simulink library "socmemlib"  (R2021a)
settings: Solver=VariableStepAuto  StartTime=0.0  StopTime=10.0  RelTol=1e-3
PreLoadFcn:
  | soc.internal.HWSWMessageTypeDef();
  | hsb.blkcb2.defineTypes;
undefined symbols (not defined in the file or in its folder): BurstRequest2BusObj, gcbh, hsb, m, ReadAccessBusObj, rearb, RegA, sendFifoFreeMsg, soc, WriteAccessBusObj
libraries: socmemlib_internal x59, priv_hsblib_beta2 x34, socsharedlib_internal x2, socqueuelib_internal x1, simulink x1
(part 4 of 5)

== stateflow chart socmemlib/Memory Channel/Writer 1/To Memory Channel/Addressable To Memory Channel/Addressable Channel Write Slave Interface/A4M Wr Slave BFM ==
  settings: updateMethod=DISCRETE  sampleTime=ChFrameSampleTime  enableNonTerminalStates=1
  state fullchart
    state requestPipeline [parallel]
      settings: executionOrder=2
      state waitForTransaction
        entry:
        wrCtrlS2M.wr_ready = true;
      state queueTransaction
        entry:
        checkAddressRange(double(wrCtrlM2S.wr_addr),double(wrCtrlM2S.wr_len), ...
        MRRegionSize,'Writer',ChTDATAWidth);
        FIFOChGatherCount = wrCtrlM2S.wr_len/ChLength;
        ReqFIFO.data = wrCtrlM2S;
        send(ReqFIFO);
        transInFlight = transInFlight +1;
      state waitForValid
      state readyTrue
        entry:
        wrCtrlS2M.wr_ready = true;
      state queueData
        entry:
        DataFIFO.data = packDataIn;
        send(DataFIFO);
        dataInFlight = dataInFlight +1;
        FIFOGatheredCount = FIFOGatheredCount+1;
      state waitForDataFIFO
      state waitFor1cycle
      state readyFalse1
        entry:
        wrCtrlS2M.wr_ready = false;
      state readyFalse
        entry:
        wrCtrlS2M.wr_ready = false;
      state queueLastData
        entry:
        if (wrCtrlM2S.wr_valid == true) && ...
        (dataInFlight<PipelineDepth+1)
        DataFIFO.data = packDataIn;
        send(DataFIFO);
        dataInFlight = dataInFlight +1;
        FIFOGatheredCount = FIFOGatheredCount+1;
        end
      state waitForFIFOs
      (default) -> waitForTransaction
      waitForFIFOs -> waitForTransaction : [(transInFlight<PipelineDepth) && ...
          |  (dataInFlight<PipelineDepth)]
      waitFor1cycle -> waitForTransaction [order 2] : after(ChFrameSampleTime, sec)
      waitForTransaction -> queueTransaction : [wrCtrlM2S.wr_valid == true]
      waitForValid -> queueData : [wrCtrlM2S.wr_valid == true]
      readyTrue -> waitForValid : after(ChFrameSampleTime, sec)
      queueTransaction -> queueData : {FIFOGatheredCount = 0;}
      queueData -> readyTrue [order 3]
      waitForDataFIFO -> readyTrue : [dataInFlight<PipelineDepth]
      queueData -> waitFor1cycle [order 1] : [(FIFOGatheredCount == FIFOChGatherCount)]
      queueData -> readyFalse1 [order 2] : [~(dataInFlight<PipelineDepth)]
      queueLastData -> waitFor1cycle [order 1] : [(FIFOGatheredCount == FIFOChGatherCount)]
      queueLastData -> waitForDataFIFO [order 2]
      waitFor1cycle -> readyFalse [order 1] : [~((transInFlight<PipelineDepth) && ...
          |  (dataInFlight<PipelineDepth))]
      readyFalse1 -> queueLastData : after(ChFrameSampleTime, sec)
      readyFalse -> waitForFIFOs : after(ChFrameSampleTime, sec)
    state initVars [parallel]
      settings: executionOrder=1
      state init
        entry:
        wrCtrlS2M = struct('wr_ready', true, 'wr_bvalid', false, 'wr_complete', false);
        locBData = zeros(4096,1,'uint8'); % FIXME: 4096 is absolute max size; MaximumBurstSize reflects tdata/len
        gatherBuffer = zeros(ChGatherBufferSize, 1, 'uint8');
        gatherBufferIndex = 1;
        burstsInFlight = 0;
        transInFlight = 0;
        dataInFlight = 0;
        frameDone = false;
      (default) -> fullchart.initVars.init
    state sendRequests [parallel]
      settings: executionOrder=3
      state waitForReq
        entry:
      state addrAndFirstData
        entry:
        CurrReq = ReqFIFO.data;
        locBAddr = double(CurrReq.wr_addr);
        [locChGatherCount, nthBSize, locChGatherBufferBurstCount] = ...
        calcDerivedInfo(double(CurrReq.wr_len), ChLength, ChTDATAWidth, ...
        ChFrameGatherBufferSize,  ChGatherBufferSize);
      state gather
        entry:
        CurrData = DataFIFO.data;
        gatheredCount = gatheredCount+1;
        gatherBuffer(gatherBufferIndex:gatherBufferIndex+ChFrameGatherBufferSize-1) = CurrData;
        gatherBufferIndex = gatherBufferIndex + ChFrameGatherBufferSize;
        dataInFlight = dataInFlight - 1;
      state waitForData
      state waitForAllBurstsToComplete
      note: If we are at the last burst OR we have enough data for one or more max-sized bursts
      state createBurst
        entry:
        if sentBurstCount == (locChGatherBufferBurstCount-1)
        currBSize = nthBSize;
        else
        currBSize = MaximumBurstSize;
        end
        burstNum = burstNum+1;
        locBData(1:currBSize) = gatherBuffer(sentBufferIndex:sentBufferIndex+currBSize-1);
      state sendBurst
        entry:
        writeToMem.data = struct('accessID', burstNum, ...
        'addr', locBAddr, 'size', currBSize,  ...
        'wdata', locBData, 'bufferAction', BufferAction.none);
        send(writeToMem);
        sentBufferIndex = sentBufferIndex + currBSize;
        locBAddr = locBAddr + currBSize;
        sentBurstCount = sentBurstCount+1;
        burstsInFlight = burstsInFlight + 1;
        if sentBurstCount == locChGatherBufferBurstCount
        frameDone=true;
        end
      (default) -> waitForReq
      waitForAllBurstsToComplete -> waitForReq : [burstsInFlight==0]
          | {transInFlight = transInFlight -1;}
      waitForReq -> addrAndFirstData : ReqFIFO
      addrAndFirstData -> gather : DataFIFO
          | { gatherBufferIndex = 1;sentBurstCount = 0; gatheredCount = 0; }
      waitForData -> gather : DataFIFO
      (junction 348) -> waitForAllBurstsToComplete [order 2] : [sentBurstCount == locChGatherBufferBurstCount]
      gather -> waitForData [order 2]
      (junction 348) -> waitForData [order 3] : [gatheredCount < locChGatherCount]
          | { gatherBufferIndex = 1;}
      gather -> createBurst [order 1] : [(gatheredCount == locChGatherCount) || (rem(gatherBufferIndex-1,MaximumBurstSize)==0)]
          | { sentBufferIndex = 1;}
      (junction 348) -> createBurst [order 1] : [sentBufferIndex < gatherBufferIndex]
      sendBurst -> (junction 348) : [burstsInFlight < InterconnectDepth]
      createBurst -> sendBurst : [memReady]
    state BurstsHandler [parallel]
      settings: executionOrder=4
      state init
        entry:
        wrCtrlS2M.wr_bvalid = false;
        wrCtrlS2M.wr_complete = false;
      state sendFrame
      state sendBursts
      state waitforFrameComplete
      state waitforBurstDone
        entry:
        wrCtrlS2M.wr_bvalid = false;
        wrCtrlS2M.wr_complete = true;
      state waitfor1Clock
      state writeIsDone
        entry:
        burstsInFlight=0;
        frameDone=false;
        wrCtrlS2M.wr_bvalid = true;
        wrCtrlS2M.wr_complete = true;
      state burstIsDone
        entry:
        if burstsInFlight >0
        wrCtrlS2M.wr_bvalid = true;
        burstsInFlight = burstsInFlight - 1;
        end
      state frameIsDone
        entry:
        if frameDone
        wrCtrlS2M.wr_complete = true;
        frameDone = false;
        end
      (default) -> fullchart.BurstsHandler.init
      (junction 413) -> fullchart.BurstsHandler.init [order 2]
      (junction 424) -> fullchart.BurstsHandler.init [order 2]
      fullchart.BurstsHandler.init -> sendFrame [order 1] : [frameDone && (ChLength>1)]
      fullchart.BurstsHandler.init -> sendBursts [order 2] : [burstsInFlight>0 || frameDone]
      (junction 424) -> waitforBurstDone [order 1] : [burstsInFlight>0]
      sendFrame -> waitforFrameComplete : after(ChFrameSampleTime,sec)
      sendBursts -> waitforBurstDone : after(ChFrameSampleTime,sec)
      waitfor1Clock -> waitforBurstDone : after(ChFrameSampleTime,sec)
      waitforFrameComplete -> writeIsDone : [memReady]
      waitforBurstDone -> burstIsDone : [memReady]
      frameIsDone -> (junction 424) : after(ChFrameSampleTime,sec)
      (junction 413) -> writeIsDone [order 1] : [frameDone && memReady]
      burstIsDone -> waitfor1Clock [order 1] : [burstsInFlight>0]
      writeIsDone -> (junction 413) : after(ChFrameSampleTime,sec)
      burstIsDone -> frameIsDone [order 2]
  (default) -> fullchart
  data: varargin function_input; varargout function_output; varargin function_input; packDataIn input; writeToMem output Bus: WriteAccessBusObj; wrCtrlS2M output Bus: WriteControlS2MBusObj; gatherBufferIndex local =1; burstNum local =0; gatherBuffer local; sentBurstCount local =0; gatheredCount local =0; locBData local uint8; ChFrameSampleTime parameter; locChGatherBufferBurstCount local; locChGatherCount local; ChFrameGatherBufferSize parameter; MaximumBurstSize parameter; ChLength parameter; ChTDATAWidth parameter; nthBSize local; locBAddr local; wrCtrlM2S input Bus: WriteControlM2SBusObj; ChGatherBufferSize parameter; memReady input; currBSize local; sentBufferIndex local; MRRegionSize parameter; PipelineDepth parameter; InterconnectDepth parameter; burstsInFlight local =0; ReqFIFO local Bus: WriteControlM2SBusObj; CurrReq local Bus: WriteControlM2SBusObj; DataFIFO local; CurrData local; FIFOChGatherCount local; FIFOGatheredCount local =0; transInFlight local =0; dataInFlight local =0; frameDone local =false
  function varargout = calcDerivedInfo(varargin):
    | function varargout = calcDerivedInfo(varargin)
    |     [varargout{1:nargout}] = hsb.blkcb2.PUPCodegenCb('calcDerivedInfo',varargin{:});
    | end
  function checkAddressRange(varargin):
    | function checkAddressRange(varargin)
    | 
    |     hsb.blkcb2.PUPCodegenCb('checkAddressRange',varargin{:});
    |     
    | end

== stateflow chart socmemlib/Memory Channel/Writer 1/To Memory Channel/Addressable To Memory Channel/Addressable Channel Write Slave Interface/Chart ==
  settings: updateMethod=DISCRETE  sampleTime=ChFrameSampleTime
  state init
    entry:
    readyDiscrete = true;
  state notvalid
    entry:
    readyDiscrete = false;
  (default) -> init
  notvalid -> init [order 1] : [readyFiM==true]
  init -> notvalid : [readyFiM==false]
  notvalid -> notvalid [order 2] : [readyFiM==false]
  data: readyFiM input; readyDiscrete output

== stateflow chart socmemlib/Memory Channel/Writer 1/To Memory Channel/Software Streaming To Memory Channel/Channel Streaming Slave Interface/A4S BFM ==
  settings: enableNonTerminalStates=1
  state fullchart
    state workChart [parallel]
      settings: executionOrder=1
      state init
        entry:
        gatherBuffer = zeros(ChGatherBufferSize, 1, 'uint8');
        bdata = zeros(MaximumBurstSize,1,'uint8');
      state requestBuffer
        entry:
        bdata = zeros(MaximumBurstSize,1,'uint8');
        MsgReqCtrl(); % Request a buffer
        writeToMem.data = struct('accessID', 0, 'addr', NO_INFLOW_DELAY, 'size', 0,  ...
        'wdata', bdata, 'bufferAction', BufferAction.request , ...
        'timingMode', TimingMode.untimed);
        send(writeToMem);
      state waitForEvent
      state gather
        entry:
        [packDataIn,valid] = MsgRecvCtrl();
        if valid
        gatheredCount = gatheredCount+1;
        gatherBuffer(gatherBufferIndex:gatherBufferIndex+ChFrameGatherBufferSize-1) = packDataIn;
        gatherBufferIndex = gatherBufferIndex + ChFrameGatherBufferSize;
        end
      state nextGather
      state sendBursts
        entry:
        reqAddr = NO_INFLOW_DELAY;
        burstNum = burstNum+1;
        bdata(1:BurstSize) = gatherBuffer(gatherBufferIndex:gatherBufferIndex+BurstSize-1);
        if sentBurstCount == ChGatherBufferBurstCount - 1;
        bufferAction = BufferAction.release;
        else
        bufferAction = BufferAction.none;
        end
        writeToMem.data = struct('accessID', burstNum, 'addr', reqAddr, 'size', BurstSize,  ...
        'wdata', bdata, 'bufferAction', bufferAction, 'timingMode', TimingMode.untimed);
        send(writeToMem);
        gatherBufferIndex = gatherBufferIndex + BurstSize;
        sentBurstCount = sentBurstCount+1;
      (default) -> init
      init -> requestBuffer
      nextGather -> requestBuffer [order 2]
      requestBuffer -> waitForEvent
      (junction 40) -> waitForEvent [order 2]
      waitForEvent -> gather : event
      nextGather -> gather [order 1] : event
      (junction 43) -> nextGather [order 1] : [sentBurstCount == ChGatherBufferBurstCount] { gatherBufferIndex = 1; sentBurstCount = 0; }
      gather -> (junction 40) : after(0,sec)
      (junction 40) -> sendBursts [order 1] : [gatheredCount == ChGatherCount] { gatherBufferIndex = 1; gatheredCount = 0; }
      (junction 43) -> sendBursts [order 2]
      sendBursts -> (junction 43) : after(0,sec)
  note: NOTE: Trying to use junctions instead
      | of state for 'nextGather' resulted in some
      | funky back-tracing where both transitions of
      | junction outputs were executed.
  (default) -> fullchart
  data: writeToMem output Bus: WriteAccessBusObj; packDataIn local; valid local boolean =false; bdata local uint8; burstNum local =0; BurstSize parameter; ChFrameGatherBufferSize parameter; ChGatherBufferBurstCount parameter; ChGatherBufferSize parameter; ChGatherCount parameter; gatherBuffer local; gatherBufferIndex local =1; gatheredCount local =0; MaximumBurstSize parameter; NO_INFLOW_DELAY constant double =-2; bufferAction local Enum: BufferAction; reqAddr local; sentBurstCount local =0; event input Bus: rteEvent

== stateflow chart socmemlib/Memory Channel/Writer 1/To Memory Channel/Streaming To Memory Channel/Channel Streaming Slave Interface/A4S BFM ==
  settings: updateMethod=DISCRETE  sampleTime=ChFrameSampleTime  enableNonTerminalStates=1
  state init
    entry:
    gatherBuffer = zeros(ChGatherBufferSize, 1, 'uint8');
    bdata = zeros(MaximumBurstSize,1,'uint8');
  state waitForValid
  state gather
    entry:
    gatheredCount = gatheredCount+1;
    gatherBuffer(gatherBufferIndex:gatherBufferIndex+ChFrameGatherBufferSize-1) = packDataIn;
    gatherBufferIndex = gatherBufferIndex + ChFrameGatherBufferSize;
  state nextGather
  state sendBursts
    entry:
    burstNum = burstNum+1;
    bdata(1:BurstSize) = gatherBuffer(gatherBufferIndex:gatherBufferIndex+BurstSize-1);
    if tlast
    bufferAction = BufferAction.release;
    else
    bufferAction = BufferAction.none;
    end
    writeToMem.data = struct('accessID', burstNum, 'addr', -1, 'size', BurstSize,  ...
    'wdata', bdata, 'bufferAction', bufferAction);
    send(writeToMem);
    gatherBufferIndex = gatherBufferIndex + BurstSize;
    sentBurstCount = sentBurstCount+1;
  (default) -> init
  init -> waitForValid
  nextGather -> waitForValid : after(ChFrameSampleTime, sec)
  waitForValid -> gather : [valid == true]
  gather -> nextGather [order 2]
  gather -> sendBursts [order 1] : [gatheredCount == ChGatherCount] { gatherBufferIndex = 1; gatheredCount = 0; }
  sendBursts -> nextGather [order 1] : [sentBurstCount == ChGatherBufferBurstCount] { gatherBufferIndex = 1; sentBurstCount = 0; }
  sendBursts -> sendBursts [order 2]
  data: packDataIn input; writeToMem output Bus: WriteAccessBusObj; valid input boolean; tlast input boolean; gatherBufferIndex local =1; burstNum local =0; gatherBuffer local; sentBurstCount local =0; gatheredCount local =0; bdata local uint8; BurstSize parameter; ChFrameSampleTime parameter; ChGatherBufferBurstCount parameter; ChGatherBufferSize parameter; ChGatherCount parameter; ChFrameGatherBufferSize parameter; MaximumBurstSize parameter; bufferAction local Enum: BufferAction

== stateflow chart socmemlib/Memory Channel/Writer 1/To Memory Channel/Streaming To Memory Channel/Channel Streaming Slave Interface/Chart ==
  settings: updateMethod=DISCRETE  sampleTime=ChFrameSampleTime
  state init
    entry:
    readyDiscrete = true;
  state notvalid
    entry:
    readyDiscrete = false;
  (default) -> init
  notvalid -> init [order 1] : [readyFiM==true]
  init -> notvalid : [readyFiM==false]
  notvalid -> notvalid [order 2] : [readyFiM==false]
  data: readyFiM input; readyDiscrete output

== stateflow chart socmemlib/Memory Channel/Writer 1/To Memory Channel/Streaming Video To Memory Channel/Channel Streaming Video Slave Interface/A4SV BFM ==
  settings: updateMethod=DISCRETE  sampleTime=ChFrameSampleTime  enableNonTerminalStates=1
  state fullchart
    state workChart [parallel]
      settings: executionOrder=1
      state init
        entry:
        gatherBuffer = zeros(ChGatherBufferSize, 1, 'uint8');
        bdata = zeros(MaximumBurstSize,1,'uint8');
      state waitForValid
      state gather
        entry:
        gatheredCount = gatheredCount+1;
        gatherBuffer(gatherBufferIndex:gatherBufferIndex+ChFrameGatherBufferSize-1) = packDataIn;
        gatherBufferIndex = gatherBufferIndex + ChFrameGatherBufferSize;
      state nextGather
      state sendBursts
        entry:
        burstNum = burstNum+1;
        tlast = ctrl.hEnd && ctrl.vEnd;
        if tlast
        bufferAction = BufferAction.release;
        else
        bufferAction = BufferAction.none;
        end
        bdata(1:BurstSize) = gatherBuffer(gatherBufferIndex:gatherBufferIndex+BurstSize-1);
        writeToMem.data = struct('accessID', burstNum, 'addr', -1, 'size', BurstSize,  ...
        'wdata', bdata, 'bufferAction', bufferAction);
        send(writeToMem);
        gatherBufferIndex = gatherBufferIndex + BurstSize;
        sentBurstCount = sentBurstCount+1;
      (default) -> init
      init -> waitForValid
      nextGather -> waitForValid : after(ChFrameSampleTime, sec)
      waitForValid -> gather : [ctrl.valid == true]
      gather -> nextGather [order 2]
      gather -> sendBursts [order 1] : [gatheredCount == ChGatherCount] { gatherBufferIndex = 1; gatheredCount = 0; }
      sendBursts -> nextGather [order 1] : [sentBurstCount == ChGatherBufferBurstCount] { gatherBufferIndex = 1; sentBurstCount = 0; }
      sendBursts -> sendBursts [order 2]
  note: NOTE: Trying to use junctions instead
      | of state for 'nextGather' resulted in some
      | funky back-tracing where both transitions of
      | junction outputs were executed.
  (default) -> fullchart
  data: packDataIn input; writeToMem output Bus: WriteAccessBusObj; ctrl input Bus: pixelcontrol; gatherBufferIndex local =1; burstNum local =0; gatherBuffer local; sentBurstCount local =0; gatheredCount local =0; bdata local uint8; BurstSize parameter; ChFrameSampleTime parameter; ChGatherBufferBurstCount parameter; ChGatherBufferSize parameter; ChGatherCount parameter; ChFrameGatherBufferSize parameter; MaximumBurstSize parameter; tlast local; bufferAction local Enum: BufferAction

== stateflow chart socmemlib/Memory Channel/Writer 1/To Memory Channel/Streaming Video To Memory Channel/Channel Streaming Video Slave Interface/Chart ==
  settings: updateMethod=DISCRETE  sampleTime=ChFrameSampleTime
  state init
    entry:
    readyDiscrete = true;
  state notvalid
    entry:
    readyDiscrete = false;
  (default) -> init
  notvalid -> init [order 1] : [readyFiM==true]
  init -> notvalid : [readyFiM==false]
  notvalid -> notvalid [order 2] : [readyFiM==false]
  data: readyFiM input; readyDiscrete output

== stateflow chart socmemlib/Memory Channel/Writer 1/bufDoneGate/async/Buffer Request Gate ==
  settings: enableNonTerminalStates=1
  state waitForBufDone
  state waitForFrameDone
    entry:
    forward(DoneIn, int_Done);
  state dequeue_internal
  state forwardBufDone
    entry:
    forward(int_Done, DoneOut);
  (default) -> waitForBufDone
  forwardBufDone -> waitForBufDone
  waitForBufDone -> waitForFrameDone : DoneIn
  waitForFrameDone -> dequeue_internal : BufDoneIn
  dequeue_internal -> forwardBufDone : int_Done
  data: DoneIn input boolean; BufDoneIn input; DoneOut output boolean; int_Done local boolean

== stateflow chart socmemlib/Memory Channel/Writer 1/bufReqGate/async/Buffer Request Gate ==
  settings: enableNonTerminalStates=1
  state waitForBufDone
  state waitForFrameDone
    entry:
    forward(bufReqIn, int_bufReq);
  state dequeue_internal
  state forwardBufDone
    entry:
    forward(int_bufReq, bufReqOut);
  (default) -> waitForBufDone
  waitForBufDone -> waitForBufDone [order 2] : BufGntIn
  forwardBufDone -> waitForBufDone
  waitForBufDone -> waitForFrameDone [order 1] : bufReqIn
  waitForFrameDone -> dequeue_internal : BufGntIn
  dequeue_internal -> forwardBufDone : int_bufReq
  data: bufReqIn input Bus: rteEvent; BufGntIn input; bufReqOut output Bus: rteEvent; int_bufReq local Bus: rteEvent

== stateflow chart socmemlib/Memory Traffic Generator/Generate Burst Request ==
  settings: enableNonTerminalStates=1
  state genMachine
    state MakeBurstRequests [parallel]
      settings: executionOrder=2
      state init
        entry:
        burstNum = 0;
        startTime = BurstInterAccessTimes(1);
      state INACTIVE
      state genReq
        entry:
        [accen, size] = genNextRequest(BurstSize,BurstInterAccessTimes);
      state terminate
      state waitForLocalDone
      state execReq
        entry:
        burstNum = burstNum +1;
        burstReq.data = struct('masterID',-1,'reqID', burstNum,'reqKind',MasterKindEnum.Dummy, 'port', -1, 'size', size);
        send(burstReq);
      (default) -> init
      init -> (junction 52) : after (startTime, sec)
      (junction 52) -> INACTIVE [order 1] : [TotalBurstRequests == 0]
      (junction 52) -> genReq [order 2]
      (junction 89) -> genReq [order 2]
      waitForLocalDone -> genReq : localDone
      genReq -> (junction 54) : after(0,sec)
      (junction 54) -> terminate [order 1] : [burstNum == TotalBurstRequests]
      (junction 54) -> execReq [order 2]
      (junction 89) -> waitForLocalDone [order 1] : [WaitForDone==true]
      execReq -> (junction 89) : after(accen,sec)
    state HandleDones [parallel]
      settings: executionOrder=1
      state waitForDone
      state forwardDone
        entry:
        forward(burstDone, localDone);
      (default) -> waitForDone
      forwardDone -> waitForDone
      (junction 78) -> waitForDone [order 2]
      waitForDone -> (junction 78) : burstDone
      (junction 78) -> forwardDone [order 1] : [WaitForDone==true]
  data: varargout function_output; varargin function_input; accen local; size local; burstNum local; burstReq output Bus: BurstRequest2BusObj; BurstSize parameter double; TotalBurstRequests parameter; BurstInterAccessTimes parameter; startTime local; WaitForDone parameter; burstDone input Bus: BurstRequest2BusObj; localDone local Bus: BurstRequest2BusObj
  function varargout = genNextRequest(varargin):
    | function varargout = genNextRequest(varargin)
    |     [varargout{1:nargout}] = hsb.blkcb2.MemoryInterconnectControllerCodegenCb('GenDummyBurstRequest', varargin{:});
    | end

== stateflow chart socmemlib/Memory Channel/Memory Region Controller/MemRegionCtrlChart ==
  settings: enableNonTerminalStates=1
  state Initialize
    entry:
    ddinfo = zeros([5 1]);
    currWrBuf = 0;
    bufBaseAddr = calcBufBaseAddresses(RegionBaseAddress, NumBuffers, AlignedBufBoundary);
  state AddWrBuf
    entry:
    currWrBuf = currWrBuf+1;
    wrBufAvail.data = currWrBuf; % data == buffer number
    send(wrBufAvail);
  state Arbitration
    state ReadArbitration [parallel]
      settings: executionOrder=1
      state WaitForRdReq
      state WaitForRdBuf
        entry:
        ddinfo(1:2) = [rdReq.data.reqID, double(length(rdBufAvail))];
        ddlogger(2, DDEvent2.BufRequest, ddinfo);
        forward(rdReq, int_rdReq);
      state RdGnt1
        entry:
        currRdBuf = rdBufAvail.data;
      state RdGnt2
        entry:
        int_rdReq.data.state = DDEvent2.BufGrant;
        int_rdReq.data.buffID = currRdBuf;
        int_rdReq.data.buffAddr = bufBaseAddr(currRdBuf);
        ddinfo(1:3) = [currRdBuf, int_rdReq.data.buffAddr, double(length(rdBufAvail))];
        ddlogger(2, DDEvent2.BufGrant, ddinfo);
        forward(int_rdReq, rdGnt);
      state rdExecuting
        entry:
        rdBufAck.data = currRdBuf; % data == buffer number
        ddlogger(2, DDEvent2.BufExecuting, ddinfo);
        send(rdBufAck);
      (default) -> WaitForRdReq
      rdExecuting -> WaitForRdReq
      WaitForRdReq -> WaitForRdBuf : rdReq
      WaitForRdBuf -> RdGnt1 : rdBufAvail
      RdGnt1 -> RdGnt2 : int_rdReq
      RdGnt2 -> rdExecuting
    state ReadAck [parallel]
      settings: executionOrder=3
      state WaitForRdDone
        entry:
        ddinfo = [0;0;0;0;0];
        ddlogger(2, DDEvent2.BufIdle, ddinfo);
      state WaitForRdBufAck
        entry:
        %Now done in Channel to Memory Interface Reader
        %ddinfo(1:2) = [rdDone.data.reqID,double(length(rdBufAvail))];
        %ddlogger(2, DDEvent2.BufDone, ddinfo);
        forward(rdDone, int_rdDone);
      state RdGnt3
        entry:
        currRdBufAck = rdBufAck.data;
      state RdDone
        entry:
        wrBufAvail.data = currRdBufAck; % data == buffer number
        ddinfo(1:3) = [currRdBufAck, bufBaseAddr(currRdBufAck), double(length(rdBufAvail))];
        ddlogger(2, DDEvent2.BufAck, ddinfo);
        send(wrBufAvail);
      (default) -> WaitForRdDone
      RdDone -> WaitForRdDone
      WaitForRdDone -> WaitForRdBufAck : rdDone
      WaitForRdBufAck -> RdGnt3 : rdBufAck
      RdGnt3 -> RdDone : int_rdDone
    state WriteArbitration [parallel]
      settings: executionOrder=2
      state WaitForWrReq
      state WaitForWrBuf
        entry:
        ddinfo(1:2) = [wrReq.data.reqID, double(length(wrBufAvail))];
        ddlogger(1, DDEvent2.BufRequest, ddinfo);
        forward(wrReq, int_wrReq);
      state WrGnt1
        entry:
        currWrBuf = wrBufAvail.data;
      state WrGnt2
        entry:
        int_wrReq.data.state = DDEvent2.BufGrant;
        int_wrReq.data.buffID = currWrBuf;
        int_wrReq.data.buffAddr = bufBaseAddr(currWrBuf);
        ddinfo(1:3) = [currWrBuf, int_wrReq.data.buffAddr, double(length(wrBufAvail))];
        ddlogger(1, DDEvent2.BufGrant, ddinfo);
        forward(int_wrReq, wrGnt);
      state wrExecuting
        entry:
        wrBufAck.data = currWrBuf; % data == buffer number
        ddlogger(1, DDEvent2.BufExecuting, ddinfo);
        send(wrBufAck);
      (default) -> WaitForWrReq
      wrExecuting -> WaitForWrReq
      WaitForWrReq -> WaitForWrBuf : wrReq
      WaitForWrBuf -> Arbitration.WriteArbitration.WrGnt1 : wrBufAvail
      Arbitration.WriteArbitration.WrGnt1 -> WrGnt2 : int_wrReq
      WrGnt2 -> wrExecuting
    state WriteAck [parallel]
      settings: executionOrder=4
      state WaitForWrDone
        entry:
        ddinfo = [0;0;0;0;0];
        ddlogger(1, DDEvent2.BufIdle, ddinfo);
      state WaitForWrBufAck
        entry:
        % Now done in Channel to Memory Interface Writer
        %ddinfo(1:2) = [wrDone.data.reqID,double(length(wrBufAvail))];
        %ddlogger(1, DDEvent2.BufDone, ddinfo);
        forward(wrDone, int_wrDone);
      state WrGnt1
        entry:
        currWrBufAck = wrBufAck.data;
      state WrDone
        entry:
        rdBufAvail.data = currWrBufAck; % data == buffer number
        ddinfo(1:3) = [currWrBufAck, bufBaseAddr(currWrBufAck), double(length(wrBufAvail))];
        ddlogger(1, DDEvent2.BufAck, ddinfo);
        send(rdBufAvail);
      (default) -> WaitForWrDone
      WrDone -> WaitForWrDone
      WaitForWrDone -> WaitForWrBufAck : wrDone
      WaitForWrBufAck -> Arbitration.WriteAck.WrGnt1 : wrBufAck
      Arbitration.WriteAck.WrGnt1 -> WrDone : int_wrDone
  (default) -> Initialize
  Initialize -> AddWrBuf : after(1e-12, sec) % FIXME
  (junction 63) -> AddWrBuf [order 1] : [currWrBuf < NumBuffers]
  AddWrBuf -> (junction 63) : after(1e-12,sec) % FIXME
  (junction 63) -> Arbitration [order 2]
  data: varargin function_input; varargout function_output; wrReq input Bus: BufferRequest2BusObj; wrDone input Bus: BufferRequest2BusObj; rdReq input Bus: BufferRequest2BusObj; AlignedBufBoundary parameter; NumBuffers parameter; RegionBaseAddress parameter; bufBaseAddr local size=NumBuffers; currRdBuf local; currWrBuf local; wrGnt output Bus: BufferRequest2BusObj size=1; rdGnt output Bus: BufferRequest2BusObj size=1; rdBufAvail local; wrBufAvail local; int_wrReq local Bus: BufferRequest2BusObj; int_rdReq local Bus: BufferRequest2BusObj; ddinfo local; currRdBufAck local; rdBufAck local; rdDone input Bus: BufferRequest2BusObj; int_rdDone local Bus: BufferRequest2BusObj; int_wrDone local Bus: BufferRequest2BusObj; wrBufAck local; currWrBufAck local
  function varargout = calcBufBaseAddresses(varargin):
    | function varargout = calcBufBaseAddresses(varargin)
    |     [varargout{1:nargout}] = hsb.blkcb2.MemoryRegionControllerCodegenCb('calcBufBaseAddresses', varargin{:});
    | end

== stateflow chart socmemlib/Memory Traffic Generator/Request Queue with Drops/FIFO with Drops/FIFO with Drops ==
  settings: enableNonTerminalStates=1
  state top
    state inputQueueing [parallel]
      settings: executionOrder=1
      state initin
        entry:
        fifoStatusMsg.data(1:end) = fifoStatus(0,0);
      state fwdIfNotFull
        entry:
        currEntries = length(int_transaction);
        if currEntries < FIFODepth
        forward(transactionIn, int_transaction);
        currEntries = currEntries+1;
        overflowFlag = 0;
        else
        % DROP DATA
        overflowFlag = 1;
        end
      state outputFullnessMore
        entry:
        fifoStatusMsg.data(1:end) = fifoStatus(currEntries, overflowFlag);
        send(fifoStatusMsg);
      (default) -> initin
      initin -> fwdIfNotFull : transactionIn
      fwdIfNotFull -> outputFullnessMore
      outputFullnessMore -> fwdIfNotFull : transactionIn
    state outputSend [parallel]
      settings: executionOrder=2
      state initout
      state firstBurst
        entry:
        forward(int_transaction, transactionOut);
      state outputFullnessLess
        entry:
        currEntries = length(int_transaction);
        fifoStatusMsg.data(1:end) = fifoStatus(currEntries,0);
        send(fifoStatusMsg);
      state waitForBurst
      state downstreamUnblocked
        entry:
        forward(int_transaction, transactionOut);
      (default) -> initout
      initout -> firstBurst : int_transaction
      firstBurst -> outputFullnessLess
      outputFullnessLess -> waitForBurst : downstreamEmpty % emptyEvent
      downstreamUnblocked -> outputFullnessLess
      waitForBurst -> downstreamUnblocked : int_transaction
  (default) -> top
  data: out function_output; num function_input; ov function_input; transactionOut output FIFOTransactionType; transactionIn input FIFOTransactionType; int_transaction local FIFOTransactionType; downstreamEmpty input; fifoStatusMsg output =zeros([1 6]); FIFODepth parameter; FIFOAFullDepth parameter; currEntries local; overflowFlag local
  function out = fifoStatus(num,ov):
    | function out = fifoStatus(num,ov)
    | 
    | % the 'length' function doesn't seem to work inside this function
    | %num = length(int_transaction);
    | e = double(num == 0);
    | f = double(num == FIFODepth);
    | a = double(num >= FIFOAFullDepth);
    | o = ov;
    | u = 0; % cannot happen in our system
    | 
    | out = [num,e,f,a,o,u];
    | 
    | end

== stateflow chart socmemlib/Memory Channel/Reader 1/From Memory Channel/Streaming From Memory Channel/Channel Streaming Master Interface/A4S Master BFM ==
  settings: updateMethod=DISCRETE  sampleTime=ChFrameSampleTime  enableNonTerminalStates=1
  state fullchart
    state workChart1 [parallel]
      settings: executionOrder=1
      state init
        entry:
        RdReqInFlight = 0;
      state waitForReqFIFO
      state sendRdRequests
        entry:
        burstNum = burstNum+1;
        reqAddr = -1;
        %First burst of every frame must untimed
        if  (ChGatherBufferBurstCount > 1) && (mod(burstNum,ChGatherBufferBurstCount) == 1)
        reqAddr = NO_INFLOW_DELAY;
        end
        readFromMem.data = struct('accessID', burstNum, 'addr', reqAddr, 'size', BurstSize);
        send(readFromMem);
        RdReqInFlight = RdReqInFlight + 1;
      (default) -> fullchart.workChart1.init
      fullchart.workChart1.init -> waitForReqFIFO
      waitForReqFIFO -> sendRdRequests : [RdReqInFlight < FIFOAFullDepth]
      sendRdRequests -> waitForReqFIFO [order 1] : [RdReqInFlight >= FIFOAFullDepth]
      sendRdRequests -> sendRdRequests [order 2]
    state workChart2 [parallel]
      settings: executionOrder=2
      state init
        entry:
        packDataOut = zeros(ChFrameGatherBufferSize, 1, 'uint8');
        rdCtrlM2S.valid = false;
        rdCtrlM2S.tlast = false;
      state newFrame
        entry:
        gatherBuffer = zeros(ChGatherBufferSize, 1, 'uint8');
      state drivenotvalid
        entry:
        rdCtrlM2S.valid = false;
        rdCtrlM2S.tlast = false;
      state nextGather
      state gather
        entry:
        gatherBuffer(gatherBufferIndex:gatherBufferIndex+BurstSize-1) = rdResult.data.rdata(1:rdResult.data.size);
        gatherBufferIndex = gatherBufferIndex + BurstSize;
        gatheredCount = gatheredCount+1;
        RdReqInFlight = RdReqInFlight - 1;
      state driveValidData
        entry:
        gatheredCount = gatheredCount+1;
        packDataOut(1:end) = gatherBuffer(gatherBufferIndex:gatherBufferIndex+ChFrameGatherBufferSize-1);
        gatherBufferIndex = gatherBufferIndex + ChFrameGatherBufferSize;
        if (tlastCount == ChTLASTCount)
        rdCtrlM2S.valid = true;
        rdCtrlM2S.tlast = true;
        tlastCount = 1;
        else
        rdCtrlM2S.valid = true;
        rdCtrlM2S.tlast = false;
        tlastCount = tlastCount+1;
        end
      state waitForClock
      state waitForReady
        entry:
        rdCtrlM2S.valid = false;
        rdCtrlM2S.tlast = false;
      (default) -> fullchart.workChart2.init
      fullchart.workChart2.init -> newFrame
      nextGather -> newFrame : after(ChFrameSampleTime,sec)
      newFrame -> gather [order 1] : rdResult
      newFrame -> drivenotvalid [order 2]
      drivenotvalid -> gather : rdResult
      gather -> drivenotvalid [order 3]
      gather -> gather [order 2] : rdResult
      driveValidData -> nextGather [order 1] : [gatheredCount == ChGatherCount] { gatherBufferIndex = 1; gatheredCount = 0; }
      gather -> (junction 110) [order 1] : [gatheredCount == ChGatherBufferBurstCount] { gatherBufferIndex = 1; gatheredCount = 0; }
      (junction 110) -> driveValidData [order 1] : [ready == true]
      (junction 110) -> waitForReady [order 2]
      waitForReady -> driveValidData : [ready == true]
      (junction 123) -> driveValidData [order 1] : [ready == true]
      driveValidData -> waitForClock [order 2]
      (junction 123) -> waitForReady [order 2]
      waitForClock -> (junction 123) : after(ChFrameSampleTime, sec)
  (default) -> fullchart
  data: ready input boolean; readFromMem output Bus: ReadAccessBusObj; packDataOut output uint8 size=ChFrameGatherBufferSize; rdResult input Bus: ReadAccessBusObj; BurstSize parameter; ChFrameGatherBufferSize parameter; ChFrameSampleTime parameter; ChGatherBufferBurstCount parameter; ChGatherBufferSize parameter; ChGatherCount parameter; ChTLASTCount parameter; burstNum local =0; gatherBuffer local; gatherBufferIndex local =1; gatheredCount local =0; RdReqInFlight local =0; tlastCount local =1; rdCtrlM2S output Bus: StreamM2SBusObj; FIFOAFullDepth parameter; NO_INFLOW_DELAY constant double =-2; reqAddr local

== stateflow chart socmemlib/Memory Channel/Memory Region Storage/Discrete-Event Chart ==
  settings: enableNonTerminalStates=1
  state init
    entry:
    zeroRdData = zeros(MaximumAccessSize,1,'uint8');
    rdData = zeroRdData;
    zeroWrData = zeros(MaximumAccessSize, 1, 'uint8');
    log_wrData = zeroWrData;
  state WaitForFirstAccess
  state ReadData
    entry:
    log_rdAddr = rdFromMem.data.addr;
    log_rdSize = rdFromMem.data.size;
    rdStartAddr = log_rdAddr+1;
    rdEndAddr = log_rdAddr+log_rdSize;
    % feature controlled: verify( false);
    checkAddressRange(checkEnabled, rdStartAddr, rdEndAddr,log_rdSize);
    rdData(1:log_rdSize) = MemRegionDataStore(rdStartAddr:rdEndAddr);
    log_rdData = rdData;
    rdFromMem.data.rdata = rdData;
    forward(rdFromMem, rdResult);
  state WriteData
    entry:
    log_wrAddr = wrToMem.data.addr;
    log_wrSize = wrToMem.data.size;
    wrStartAddr = log_wrAddr+1;
    wrEndAddr = log_wrAddr+log_wrSize;
    checkAddressRange(checkEnabled, wrStartAddr, wrEndAddr,log_wrSize);
    log_wrData(1:log_wrSize) = wrToMem.data.wdata(1:log_wrSize);
    MemRegionDataStore(wrStartAddr:wrEndAddr) = log_wrData(1:log_wrSize);
  (default) -> init
  init -> WaitForFirstAccess
  WaitForFirstAccess -> ReadData [order 2] : rdFromMem
  (junction 8) -> WaitForFirstAccess
  WaitForFirstAccess -> WriteData [order 1] : wrToMem
  WriteData -> (junction 8)
  ReadData -> (junction 8)
  data: varargin function_input; rdResult output Bus: ReadAccessBusObj; wrToMem input Bus: WriteAccessBusObj; MemRegionDataStore data_store_memory; rdFromMem input Bus: ReadAccessBusObj; zeroRdData local; log_rdAddr local; log_rdData local; log_rdSize local [0..]; log_wrAddr local; log_wrData local; log_wrSize local; rdData local; zeroWrData local; MaximumAccessSize parameter; rdEndAddr local; rdStartAddr local; wrEndAddr local; wrStartAddr local; checkEnabled constant boolean =false
  function checkAddressRange(varargin):
    | function checkAddressRange(varargin)
    | 
    |     hsb.blkcb2.MemoryRegionControllerCodegenCb('checkAddressRange',varargin{:});
    | 
    | end

== stateflow chart socmemlib/Memory Channel/Reader 1/From Memory Channel/Addressable From Memory Channel/Addressable Channel Read Slave Interface/A4M Rd Slave BFM ==
  settings: updateMethod=DISCRETE  sampleTime=ChFrameSampleTime  enableNonTerminalStates=1
  note: Some names given during writer development. Translation to reader side.
      | *Really* might want to change these names!
      | gatherBuffer == buffer used to drive samples to the channel interface
      | gatheredCount == count of sent channel interface frames from gatherBuffer
      | locChGatherCount == total count of ch i/f frames for current transaction
      | sdaf
      |
      | Overall process:
      | make burst requests as long as pipelining/FIFOing allow
      | if this s/m cannot service results, will back up into FIFO
      | as result comes, add to gatherBuffer
      | as soon as >=1 channel frame of data is ready, start DRIVING data
      | if have reached end of current contents in gather buffer, go back and get more
      | otherwise, get next channel frame chunk of data and DRIVE it
      | DO NOT NEED to track current transaction since responses are per data xfer
      | there is nothing in protocol to indicate end of frame.
  state fullchart
    state initVars [parallel]
      settings: executionOrder=1
      state init
        entry:
        rdCtrlS2M = struct('rd_aready', true, 'rd_dvalid', false);
        packDataOut = zeros(ChFrameGatherBufferSize, 1, 'uint8');
        gatherBuffer = zeros(ChGatherBufferSize, 1, 'uint8');
        gatherBufferIndex = 1;
        burstsInFlight = 0;
        transInFlight = 0;
      (default) -> init
    state recvAndDriveData [parallel]
      settings: executionOrder=4
      state waitForResult
      state drivenotvalid
        entry:
        rdCtrlS2M.rd_dvalid = false;
      state WaitForResult1
      state resultIntoGatherBuffer
        entry:
        locBSize = rdResult.data.size;
        gatherBuffer(gatherBufferIndex:gatherBufferIndex+locBSize-1) = rdResult.data.rdata(1:locBSize);
        gatherBufferIndex = gatherBufferIndex + locBSize;
        burstsInFlight = burstsInFlight - 1;
      state nextGather
      state waitForReady
        entry:
        rdCtrlS2M.rd_dvalid = false;
      state driveValidData
        entry:
        rdCtrlS2M.rd_dvalid = true;
        packDataOut(1:end) = gatherBuffer(drivenBufferIndex:drivenBufferIndex+ChFrameGatherBufferSize-1);
        drivenBufferIndex = drivenBufferIndex + ChFrameGatherBufferSize;
      (default) -> waitForResult
      nextGather -> waitForResult : after(ChFrameSampleTime,sec)
      resultIntoGatherBuffer -> waitForResult [order 2]
      waitForResult -> (junction 89)
      (junction 89) -> drivenotvalid [order 2]
      drivenotvalid -> WaitForResult1 : after(ChFrameSampleTime,sec)
      (junction 89) -> resultIntoGatherBuffer [order 1] : rdResult
      WaitForResult1 -> resultIntoGatherBuffer : rdResult
      driveValidData -> nextGather [order 1] : [drivenBufferIndex == gatherBufferIndex]
          | { gatherBufferIndex = 1; }
      resultIntoGatherBuffer -> (junction 71) [order 1] : [gatherBufferIndex >= ChFrameGatherBufferSize-1]
          | { drivenBufferIndex = 1;}
      (junction 71) -> waitForReady [order 2]
      (junction 71) -> driveValidData [order 1] : [rdCtrlM2S.rd_dready == true]
      (junction 75) -> waitForReady [order 2]
      (junction 75) -> driveValidData [order 1] : [rdCtrlM2S.rd_dready == true]
      driveValidData -> (junction 75) [order 2] : after(ChFrameSampleTime,sec)
      waitForReady -> driveValidData : [rdCtrlM2S.rd_dready == true]
    state requestPipeline [parallel]
      settings: executionOrder=2
      state waitForTransaction
        entry:
        rdCtrlS2M.rd_aready = true;
      state captureTransaction
        entry:
        checkAddressRange(double(rdCtrlM2S.rd_addr),double(rdCtrlM2S.rd_len), ...
        MRRegionSize,'Reader',ChTDATAWidth);
        ReqFIFO.data = rdCtrlM2S;
        send(ReqFIFO);
        transInFlight = transInFlight +1;
      state readyFalse
        entry:
        rdCtrlS2M.rd_aready = false;
      state waitForFIFO
      (default) -> waitForTransaction
      waitForFIFO -> waitForTransaction : [transInFlight<PipelineDepth]
      (junction 194) -> waitForTransaction [order 2] : after(ChFrameSampleTime, sec)
      waitForTransaction -> captureTransaction : [rdCtrlM2S.rd_avalid == true]
      captureTransaction -> (junction 194)
      (junction 194) -> readyFalse [order 1] : [~(transInFlight<PipelineDepth)]
      readyFalse -> waitForFIFO : after(ChFrameSampleTime, sec)
    state sendRequests [parallel]
      settings: executionOrder=3
      state waitForReq
      state addrPhase
        entry:
        CurrReq = ReqFIFO.data;
        sentRdReqCount = 0;
        locBAddr = double(CurrReq.rd_addr);
        [locChGatherCount, nthBSize, locChGatherBufferBurstCount] = ...
        calcDerivedInfo(double(CurrReq.rd_len), ChLength, ChTDATAWidth, ...
        ChFrameGatherBufferSize, ChGatherBufferSize);
      state waitForAllBurstsToComplete
      state createRequest
        entry:
        if sentRdReqCount == locChGatherBufferBurstCount-1
        currBSize = nthBSize;
        else
        currBSize = MaximumBurstSize;
        end
        burstNum = burstNum+1;
      state SendRequest
        entry:
        readFromMem.data = struct('accessID', burstNum, 'addr', locBAddr, 'size', currBSize);
        send(readFromMem);
        locBAddr = locBAddr + currBSize;
        sentRdReqCount = sentRdReqCount + 1;
        burstsInFlight = burstsInFlight + 1;
      (default) -> waitForReq
      waitForAllBurstsToComplete -> waitForReq : [burstsInFlight==0]
          | {transInFlight = transInFlight -1;}
      waitForReq -> addrPhase : ReqFIFO
      (junction 156) -> waitForAllBurstsToComplete [order 2]
      addrPhase -> createRequest
      (junction 156) -> createRequest [order 1] : [sentRdReqCount < locChGatherBufferBurstCount]
      SendRequest -> (junction 156) : [(burstsInFlight < InterconnectDepth)]
      createRequest -> SendRequest : [memReady]
  (default) -> fullchart
  data: varargin function_input; varargout function_output; varargin function_input; readFromMem output Bus: ReadAccessBusObj; packDataOut output uint8 size=ChFrameGatherBufferSize; rdCtrlS2M output Bus: ReadControlS2MBusObj; rdResult input Bus: ReadAccessBusObj; rdCtrlM2S input Bus: ReadControlM2SBusObj; locBSize local; ChFrameGatherBufferSize parameter; ChFrameSampleTime parameter; ChGatherBufferSize parameter; ChLength parameter; gatherBuffer local; gatherBufferIndex local =1; sentRdReqCount local; ChTDATAWidth parameter; MaximumBurstSize parameter; locChGatherCount local; locBAddr local; locChGatherBufferBurstCount local; memReady input; currBSize local; nthBSize local; burstsInFlight local =0; drivenBufferIndex local; burstNum local =0; MRRegionSize parameter; ReqFIFO local Bus: ReadControlM2SBusObj size=1; CurrReq local Bus: ReadControlM2SBusObj size=1; PipelineDepth parameter double; InterconnectDepth parameter double; transInFlight local =0
  function varargout = calcDerivedInfo(varargin):
    | function varargout = calcDerivedInfo(varargin)
    |     [varargout{1:nargout}] = hsb.blkcb2.PUPCodegenCb('calcDerivedInfo',varargin{:});
    | end
  function checkAddressRange(varargin):
    | function checkAddressRange(varargin)
    | 
    |     hsb.blkcb2.PUPCodegenCb('checkAddressRange',varargin{:});
    |     
    | end

== matlab function socmemlib/Memory Channel/log/MATLAB Function ==
  data: mID input size=1; ddOut output Bus: MemChDD2BusObj; event input Enum: DDEvent2; info input size=5
function ddOut = ddlogger_mlfcn(mID, event, info)

    ddOut = hsb.blkcb2.MemoryRegionControllerCodegenCb( ...
                'DDEventLoggerLevel2', mID, event, info);

            
            
end

== stateflow chart socmemlib/Memory Channel/Reader 1/From Memory Channel/Software Streaming From Memory Channel/Channel Streaming Master Interface/A4S Master BFM ==
  settings: enableNonTerminalStates=1
  note: NOTE: Trying to use junctions instead
      | of state for 'nextGather' resulted in some
      | funky back-tracing where both transitions of
      | junction outputs were executed.
  note: NOTE: Should we make read requests either when gather buffer processed OR on a time tick?
      | If only on needed event, can combine the sendrdreq and gather sub-charts.
  state fullchart
    state workChart2 [parallel]
      settings: executionOrder=1
      state init
        entry:
        packDataOut = zeros(ChFrameGatherBufferSize, 1, 'uint8');
      note: A A gather buffer holds one or more bursts. It'll hold more than one burst when the frame size
          | is greater than one burst. This state says it needs data.
      state gatherInit
        entry:
        gatherNum = gatherNum+1;
        gatherBufferNeeded.data = gatherNum;
        send(gatherBufferNeeded);
        gatherBuffer = zeros(ChGatherBufferSize, 1, 'uint8');
        bdata = zeros(BurstSize,1,'uint8');
      note: B Iterate until have enough burst results to fill the
          | gather buffer. The 'rdResult' is coming in through
          | a message "unit delay" to avoid an algebraic loop warning.
          | (The entire message queue is synchronized to the discrete
          | time all at once.)
      state waitForResult
      state gather
        entry:
        gatherBuffer(gatherBufferIndex:gatherBufferIndex+BurstSize-1) = rdResult.data.rdata(1:rdResult.data.size);
        gatherBufferIndex = gatherBufferIndex + BurstSize;
        gatheredCount = gatheredCount+1;
      state nextGather
      note: D If the data frame size is less than the gather
          | buffer it'll iterate through this state in order to
          | not just get through data in one time step.
          | (It'll look like it just ouput the last data without this delay.)
      state waitForResult2
      note: E If the buffers are full we want to pause
          | future transfers until our consumer task has
          | drained the buffers to the target level.
      state driveDataInterval
        entry:
        error('buffer size not equal to frame size');
      state driveValidData
        entry:
        gatheredCount = gatheredCount+1;
        packDataOut(1:end)=gatherBuffer(gatherBufferIndex:gatherBufferIndex+ChFrameGatherBufferSize-1);
        gatherBufferIndex = gatherBufferIndex + ChFrameGatherBufferSize;
        MsgSendCtrl(packDataOut);
      note: C Now that we have out gather buffer, iterate until we
          | have sent it all out onto the data line.
      (default) -> fullchart.workChart2.init
      fullchart.workChart2.init -> gatherInit
      nextGather -> gatherInit
      gatherInit -> waitForResult
      waitForResult -> gather : rdResult
      gather -> (junction 129) : after(0,sec)
      waitForResult2 -> gather : rdResult
      (junction 123) -> nextGather [order 1] : [gatheredCount == ChGatherCount] { gatherBufferIndex = 1; gatheredCount = 0; }
      (junction 129) -> waitForResult2 [order 2]
      (junction 129) -> driveValidData [order 1] : [gatheredCount == ChGatherBufferBurstCount] { gatherBufferIndex = 1; gatheredCount = 0; }
      (junction 123) -> driveDataInterval [order 2]
      driveDataInterval -> driveValidData : after(0.2*ChFrameSampleTime,sec)
      driveValidData -> (junction 123) : after(0,sec)
    state workChart1 [parallel]
      settings: executionOrder=2
      state init
        entry:
        sentRdReqCount = 0;
      state sendRdRequests
        entry:
        reqAddr = NO_INFLOW_DELAY;
        burstNum = burstNum+1;
        readFromMem.data = struct('accessID', burstNum, 'addr', reqAddr, 'size', BurstSize, ...
        'rdata', zeros(4096,1,'uint8'), 'bufferAction', BufferAction.none, 'timingMode', TimingMode.untimed);
        send(readFromMem);
        sentRdReqCount = sentRdReqCount + 1;
      (default) -> fullchart.workChart1.init
      fullchart.workChart1.init -> sendRdRequests : gatherBufferNeeded
      (junction 121) -> fullchart.workChart1.init [order 1] : [sentRdReqCount == ChGatherBufferBurstCount]
      sendRdRequests -> (junction 121) : after(0,sec) % create base-event
      (junction 121) -> sendRdRequests [order 2]
  (default) -> fullchart
  data: readFromMem output Bus: ReadAccessBusObj; bdata local uint8; burstNum local =0; BurstSize parameter; ChFrameGatherBufferSize parameter; ChFrameSampleTime parameter; ChGatherBufferBurstCount parameter; ChGatherBufferSize parameter; ChGatherCount parameter; gatherBuffer local; gatherBufferIndex local =1; gatherBufferNeeded local; gatherNum local =0; gatheredCount local =0; rdResult input Bus: ReadAccessBusObj; NO_INFLOW_DELAY constant double =-2; reqAddr local; sentRdReqCount local; packDataOut local uint8 size=ChFrameGatherBufferSize

== matlab function socmemlib/Memory Controller/log/MATLAB Function ==
  data: portID input size=1; ddOut output Bus: MemCtrlDD2BusObj; event input Enum: DDEvent2; info input size=5; timestamp input; NumMasters parameter
function ddOut = ddlogger_mlfcn(portID, event, info, timestamp, NumMasters)
   
    ddOut = hsb.blkcb2.MemoryInterconnectControllerCodegenCb( ...
                'DDEventLogger2', portID, event, info, timestamp, NumMasters);

end
